simulink model "IMTrialPLL"  (R2023b)
settings: Solver=VariableStepAuto  StartTime=0.0  StopTime=16  FixedStep=10e-6  RelTol=1e-3
settings Model: Creator=Aryasetya  LastModifiedBy=Aryasetya
settings ModelReferenceCC: EnableRefExpFcnMdlSchedulingChecks=on

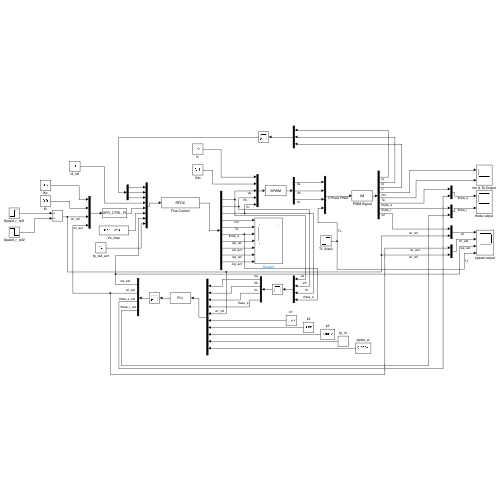
[thumbnail: Simulink's stored preview of the top-level diagram]
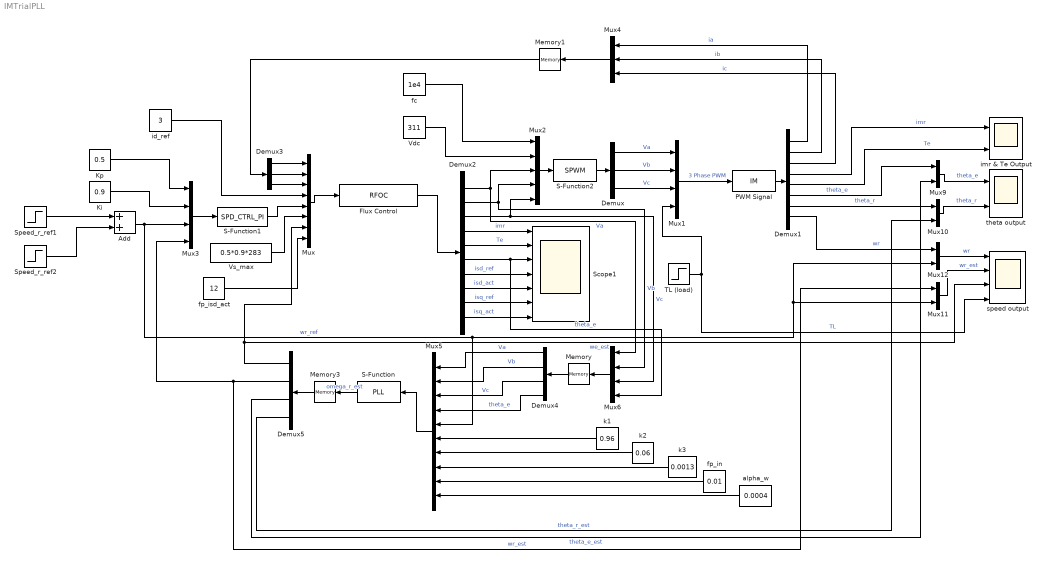
== system IMTrialPLL ==
  Add : Sum
  Demux : Demux  Outputs=3
  Demux1 : Demux  Outputs=8
  Demux2 : Demux  Outputs=10
  Demux3 : Demux  Outputs=3
  Demux4 : Demux
  Demux5 : Demux
  Flux Control : S-Function  FunctionName=RFOC  SFunctionDeploymentMode=off  EnableBusSupport=off
  Ki : Constant  Value=0.9
  Kp : Constant  Value=0.5
  Memory : Memory
  Memory1 : Memory
  Memory3 : Memory
  Mux : Mux  Inputs=8
  Mux1 : Mux
  Mux{9..12} (4 alike) : Mux  Inputs=2
  Mux2 : Mux  Inputs=5
  Mux3 : Mux
  Mux4 : Mux  Inputs=3
  Mux5 : Mux  Inputs=10
  Mux6 : Mux
  PWM Signal : S-Function  FunctionName=IM  SFunctionDeploymentMode=off  EnableBusSupport=off
  S-Function : S-Function  FunctionName=PLL  SFunctionDeploymentMode=off  EnableBusSupport=off
  S-Function1 : S-Function  FunctionName=SPD_CTRL_PI  SFunctionDeploymentMode=off  EnableBusSupport=off
  S-Function2 : S-Function  FunctionName=SPWM  SFunctionDeploymentMode=off  EnableBusSupport=off
  Scope1 : Scope  NumInputPorts=7
  Speed_r_ref1 : Step  After=50  SampleTime=0
  Speed_r_ref2 : Step  Time=10  After=-20  SampleTime=0
  TL (load) : Step  Time=5  After=3  SampleTime=0
  Vdc : Constant  Value=311
  Vs_max : Constant  Value=0.5*0.9*283
  alpha_w : Constant  Value=0.0004
  fc : Constant  Value=1e4
  fp_in : Constant  Value=0.01
  fp_isd_act : Constant  Value=12
  id_ref : Constant  Value=3
  imr & Te Output : Scope  NumInputPorts=2
  k1 : Constant  Value=0.96
  k2 : Constant  Value=0.06
  k3 : Constant  Value=0.0013
  speed output : Scope  NumInputPorts=4
  theta output : Scope  NumInputPorts=2
  wires:
  Mux1/1 -> PWM Signal/1  "3 Phase PWM"
  PWM Signal/1 -> Demux1/1
  Demux/3 -> Mux1/3  "Vc"
  Demux/2 -> Mux1/2  "Vb"
  Demux/1 -> Mux1/1  "Va"
  TL (load)/1 -> speed output/4, Mux1/4  "TL"
  Demux1/1 -> Mux4/1  "ia"
  Demux1/2 -> Mux4/2  "ib"
  Demux1/3 -> Mux4/3  "ic"
  Demux1/4 -> imr & Te Output/1  "imr"
  Demux1/5 -> imr & Te Output/2  "Te"
  Demux1/6 -> Mux9/1  "theta_e"
  Demux1/7 -> Mux10/1  "theta_r"
  Flux Control/1 -> Demux2/1
  Mux/1 -> Flux Control/1
  S-Function1/1 -> Mux/5
  Mux3/1 -> S-Function1/1
  Ki/1 -> Mux3/2
  Kp/1 -> Mux3/1
  id_ref/1 -> Mux/4
  Demux3/2 -> Mux/2
  Demux3/1 -> Mux/1
  Demux3/3 -> Mux/3
  Mux4/1 -> Memory1/1
  Memory1/1 -> Demux3/1
  Vs_max/1 -> Mux/6
  Mux2/1 -> S-Function2/1
  Demux2/1 -> Mux2/3, Mux6/1  "Va"
  Demux2/2 -> Mux2/4, Mux6/2  "Vb"
  Demux2/3 -> Mux2/5, Mux6/3  "Vc"
  S-Function/1 -> Memory3/1  "omega_r_est"
  Mux5/1 -> S-Function/1
  Memory/1 -> Demux4/1
  Demux4/2 -> Mux5/2  "Vb"
  Demux4/1 -> Mux5/1  "Va"
  Demux4/3 -> Mux5/3  "Vc"
  Demux2/4 -> Scope1/1  "imr"
  Demux2/6 -> Mux6/4, Scope1/3  "theta_e"
  Demux2/5 -> Scope1/2  "Te"
  Demux2/7 -> Scope1/4  "isd_ref"
  Demux2/8 -> Scope1/5  "isd_act"
  Demux2/9 -> Scope1/6  "isq_ref"
  Demux2/10 -> Scope1/7  "isq_act"
  Demux4/4 -> Mux5/4  "theta_e"
  Mux6/1 -> Memory/1
  S-Function2/1 -> Demux/1
  fc/1 -> Mux2/1
  Vdc/1 -> Mux2/2
  Memory3/1 -> Demux5/1
  Demux5/1 -> Mux/7, speed output/3  "we_est"
  Demux5/2 -> Mux11/1, Mux3/4  "wr_est"
  Speed_r_ref1/1 -> Add/1
  Add/1 -> Mux3/3, Mux5/5, Mux12/2, Mux11/2  "wr_ref"
  Speed_r_ref2/1 -> Add/2
  Demux1/8 -> Mux12/1  "wr"
  fp_isd_act/1 -> Mux/8
  Mux9/1 -> theta output/1  "theta_e"
  Mux10/1 -> theta output/2  "theta_r"
  Mux12/1 -> speed output/1  "wr"
  Mux11/1 -> speed output/2  "wr_est"
  Demux5/3 -> Mux9/2  "theta_e_est"
  Demux5/4 -> Mux10/2  "theta_r_est"
  k1/1 -> Mux5/6
  k2/1 -> Mux5/7
  k3/1 -> Mux5/8
  fp_in/1 -> Mux5/9
  alpha_w/1 -> Mux5/10
